simulink model "Pitch_Roll_Control"  (R2013a)
settings: Solver=ode45  StartTime=0.0  StopTime=10  MaxStep=1e-5  MinStep=1e-7  RelTol=1e-5
values from neighbouring files (symbols this model uses):
  Kd = 1/abs((DCL_Pole_1+zc)*evalfr(sys,DCL_Pole_1))    [Pitch_Roll_Controller_PD.m]    (also in Yaw_PD.m = 1/abs((DCL_Pole_1+zc)*evalfr(sys_Yaw,DCL_Pole_1)))
  Ki = T_I    [Height_Controller_PID.m]
undefined symbols (not defined in the file or in its folder): F_yIntercept, I_Theta, Kf, Kp, Motor_TimeConstant
settings Model: Creator=Ross  LastModifiedBy=Ross

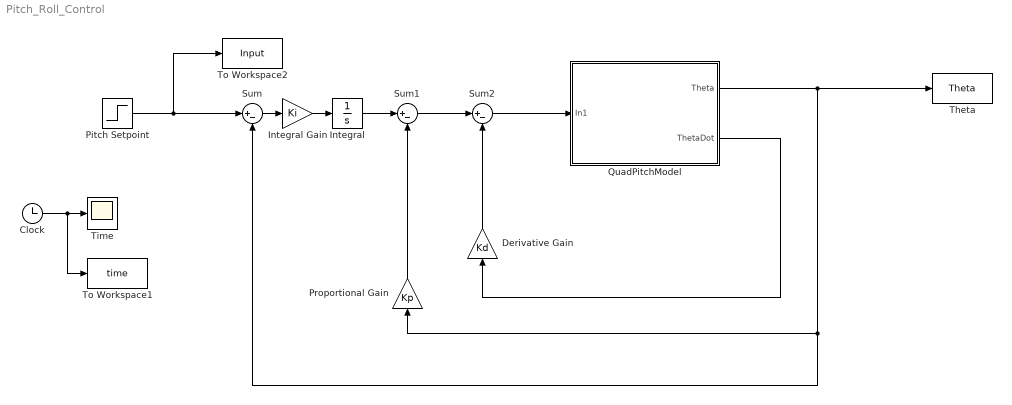
== system Pitch_Roll_Control ==
  Clock : Clock
  Derivative Gain : Gain  Gain=Kd
  Integral : Integrator
  Integral Gain : Gain  Gain=Ki
  Pitch Setpoint : Step  Time=5  SampleTime=0
  Proportional Gain : Gain  Gain=Kp
  QuadPitchModel : Subsystem
  Sum : Sum  Inputs=|+-
  Sum1 : Sum  Inputs=|+-
  Sum2 : Sum  Inputs=|+-
  Theta : ToWorkspace  VariableName=Theta  SampleTime=-1  SaveFormat=Timeseries
  Time : Scope
  To Workspace1 : ToWorkspace  VariableName=time  SampleTime=-1  SaveFormat=Timeseries
  To Workspace2 : ToWorkspace  VariableName=Input  SampleTime=-1  SaveFormat=Timeseries
  wires:
  Proportional Gain/1 -> Sum1/2
  Derivative Gain/1 -> Sum2/2
  Sum1/1 -> Sum2/1
  Integral/1 -> Sum1/1
  Integral Gain/1 -> Integral/1
  Sum/1 -> Integral Gain/1
  Clock/1 -> To Workspace1/1, Time/1
  Pitch Setpoint/1 -> Sum/1, To Workspace2/1
  Sum2/1 -> QuadPitchModel/1(In1)
  QuadPitchModel/2(ThetaDot) -> Derivative Gain/1
  QuadPitchModel/1(Theta) -> Sum/2, Proportional Gain/1, Theta/1

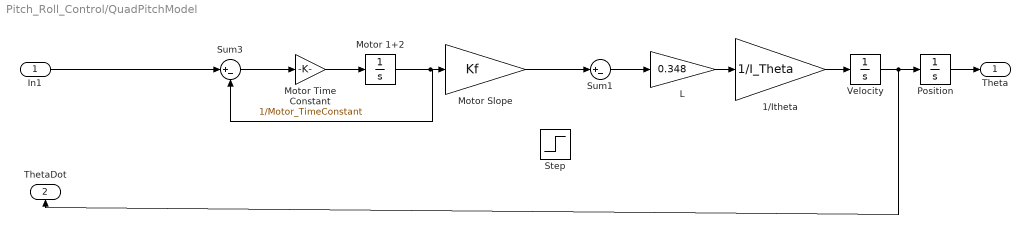
== system Pitch_Roll_Control/QuadPitchModel ==
  In1 : Inport
  1/Itheta : Gain  Gain=1/I_Theta
  L : Gain  Gain=0.348
  Motor 1+2 : Integrator
  Motor Slope : Gain  Gain=Kf
  Motor Time Constant : Gain  Gain=1/Motor_TimeConstant
  Position : Integrator
  Step : Step  Time=0  After=F_yIntercept  SampleTime=0
  Sum1 : Sum  Inputs=|+-
  Sum3 : Sum  Inputs=|+-
  Velocity : Integrator
  Theta : Outport
  ThetaDot : Outport  Port=2
  wires:
  Motor Slope/1 -> Sum1/1
  Position/1 -> Theta/1
  L/1 -> 1/Itheta/1
  Motor 1+2/1 -> Sum3/2, Motor Slope/1
  In1/1 -> Sum3/1
  Velocity/1 -> ThetaDot/1, Position/1
  Sum3/1 -> Motor Time Constant/1
  1/Itheta/1 -> Velocity/1
  Motor Time Constant/1 -> Motor 1+2/1
  Sum1/1 -> L/1
